simulink model "symulacjaZN"  (R2017b)
settings: Solver=VariableStepAuto  StartTime=0.0  StopTime=10.0  RelTol=1e-3
values from neighbouring files (symbols this model uses):
  K = 1.4    [projekt2.m]
  Kk = str2num(kin{1})    [projekt2.m]
  T1 = 1/14    (= 0.0714285714286)    [projekt2.m]
  T2 = 100    [projekt2.m]
  T3 = 10    [projekt2.m]
  T4 = 1    [projekt2.m]
settings Model: Creator=Alicja  LastModifiedBy=Alicja
settings DataIOCC: SaveFormat=Array

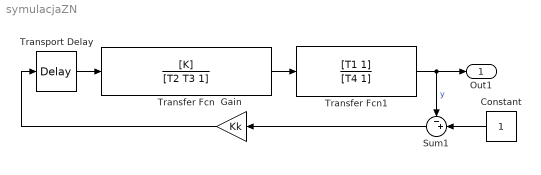
== system symulacjaZN ==
  Constant : Constant
  Gain : Gain  Gain=Kk
  Sum1 : Sum  Inputs=-+|
  Transfer Fcn : TransferFcn  Numerator=[K]  Denominator=[T2 T3 1]
  Transfer Fcn1 : TransferFcn  Numerator=[T1 1]  Denominator=[T4 1]
  Transport Delay : TransportDelay  DelayTime=20
  Out1 : Outport
  wires:
  Transport Delay/1 -> Transfer Fcn/1
  Transfer Fcn/1 -> Transfer Fcn1/1
  Gain/1 -> Transport Delay/1
  Transfer Fcn1/1 -> Out1/1, Sum1/1  "y"
  Sum1/1 -> Gain/1
  Constant/1 -> Sum1/2
